simulink model "simulation_of_simple_pendulum_motion_with_damper_winding"  (R2021a)
settings: Solver=VariableStepAuto  StartTime=0.0  StopTime=100  MaxStep=1e-3  RelTol=1e-3
settings Model: Creator=YasserNet  LastModifiedBy=YasserNet

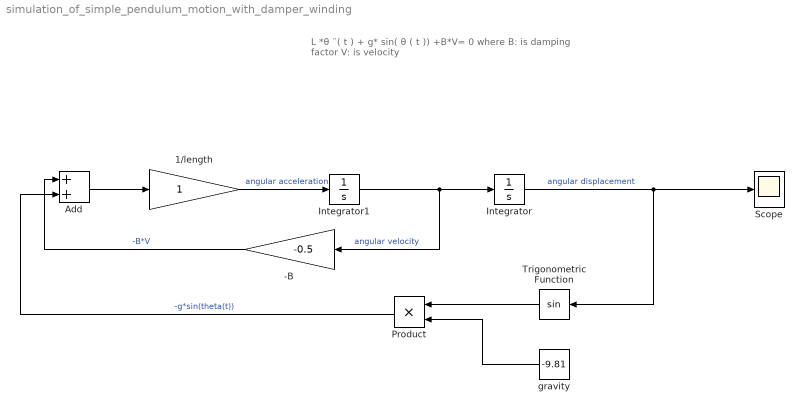
== system simulation_of_simple_pendulum_motion_with_damper_winding ==
  note: L *θ ¨( t ) + g* sin( θ ( t )) +B*V= 0
      | where B: is damping factor
      | V: is velocity
  -B : Gain  Gain=-0.5  OutDataTypeStr=double
  1/length : Gain  OutDataTypeStr=double
  Add : Sum
  Integrator : Integrator  InitialCondition=1
  Integrator1 : Integrator
  Product : Product
  Scope : Scope
  Trigonometric Function : Trigonometry
  gravity : Constant  Value=-9.81
  wires:
  Integrator/1 -> Trigonometric Function/1, Scope/1  "angular displacement"
  gravity/1 -> Product/2
  Trigonometric Function/1 -> Product/1
  1/length/1 -> Integrator1/1  "angular acceleration"
  Integrator1/1 -> Integrator/1, -B/1  "angular velocity"
  Add/1 -> 1/length/1
  -B/1 -> Add/1  "-B*V"
  Product/1 -> Add/2  "-g*sin(theta(t))"
